simulink model "blockdemo"  (Simulink 7.0)
settings: Solver=FixedStepDiscrete  StartTime=0.0  StopTime=10.0  FixedStep=1  RelTol=1e-3
InitFcn:
  | %% DSPBuilder Start
  | alt_dspbuilder_update_model(bdroot)
  | %% DSPBuilder End
libraries: allblocks_alteradspbuilder2 x12
settings Model: Creator=mjervis  LastModifiedBy=delphick
settings OptimizationCC: BlockReduction=off  BooleanDataType=off  InlineInvariantSignals=on
settings DebuggingCC: SaveWithParameterizedLinksMsg=none  SignalResolutionControl=TryResolveAllWithWarning  SolverPrmCheckMsg=none  MultiTaskDSMMsg=warning  MultiTaskCondExecSysMsg=none
settings HardwareCC: TargetUnknown=on
settings RTWCC: IncludeERTFirstTime=on
settings GRTTargetCC: TargetFcnLib=ansi_tfl_tmw.mat

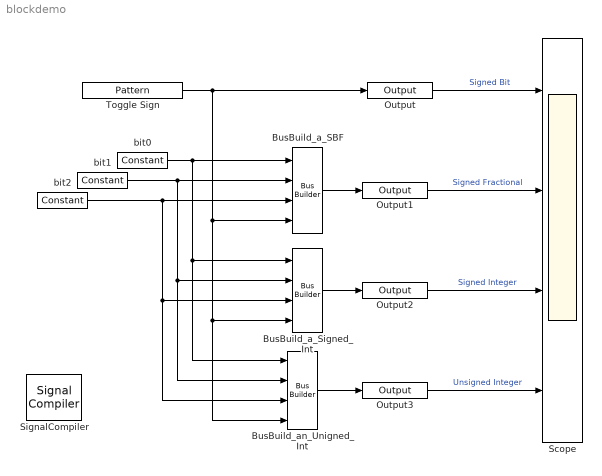
== system blockdemo ==
  BusBuild_a_SBF : allblocks_alteradspbuilder2/Bus Builder  BusType=Signed Fractional  bwl=2  bwr=2  pipeline_display=0
  BusBuild_a_Signed_Int : allblocks_alteradspbuilder2/Bus Builder  BusType=Signed Integer  bwl=4  bwr=0  pipeline_display=0
  BusBuild_an_Unigned_Int : allblocks_alteradspbuilder2/Bus Builder  BusType=Unsigned Integer  bwl=4  bwr=0  pipeline_display=0
  Output : allblocks_alteradspbuilder2/Output  iofile=C:\perforce_workspace81\main\dsp_builder2\Documentation\DesignExamples\Tutorials\UnitBlocks\IOBus\BusBuilder\tb_blockdemo\blockdemo_Output.capture  BusType=Single Bit  bwl=8  bwr=0  externalType=Inferred  PORTTYPE=Output  allowFloatingPointOverride=on  logOutputs=off
  Output1 : allblocks_alteradspbuilder2/Output  iofile=C:\perforce_workspace81\main\dsp_builder2\Documentation\DesignExamples\Tutorials\UnitBlocks\IOBus\BusBuilder\tb_blockdemo\blockdemo_Output1.capture  BusType=Signed Fractional  bwl=2  bwr=2  externalType=Inferred  PORTTYPE=Output  allowFloatingPointOverride=on  logOutputs=off
  Output2 : allblocks_alteradspbuilder2/Output  iofile=C:\perforce_workspace81\main\dsp_builder2\Documentation\DesignExamples\Tutorials\UnitBlocks\IOBus\BusBuilder\tb_blockdemo\blockdemo_Output2.capture  BusType=Signed Integer  bwl=4  bwr=0  externalType=Inferred  PORTTYPE=Output  allowFloatingPointOverride=on  logOutputs=off
  Output3 : allblocks_alteradspbuilder2/Output  iofile=C:\perforce_workspace81\main\dsp_builder2\Documentation\DesignExamples\Tutorials\UnitBlocks\IOBus\BusBuilder\tb_blockdemo\blockdemo_Output3.capture  BusType=Unsigned Integer  bwl=4  bwr=0  externalType=Inferred  PORTTYPE=Output  allowFloatingPointOverride=on  logOutputs=off
  Scope : Scope  NumInputPorts=4
      settings: YMin=-1~-2~-8~0  YMax=2~1~2~10
  SignalCompiler : allblocks_alteradspbuilder2/Signal Compiler  DeviceFamily=Stratix IV  DeviceName=AUTO  EnableSignalTap=off  SignalTapDepth=128  UseBoardBlock=off  StpUseDefaultClock=on  StpClock=Clock  ExportDir=C:\Documents and Settings\delphick\My Documents\MATLAB
  Toggle Sign : allblocks_alteradspbuilder2/Pattern  Sequence=11110000  SpecifyClock=off  use_ena=off  use_sclr=off
  bit0 : allblocks_alteradspbuilder2/Constant  mask_cst=1  BusType=Single Bit  bwl=8  bwr=0  roundMode=Truncate  satMode=Wrap  SpecifyClock=off  allowFloatingPointOverride=on  logOutputs=off  logFile=C:\perforce_workspace81\main\dsp_builder2\Documentation\DesignExamples\Tutorials\UnitBlocks\IOBus\BusBuilder\tb_blockdemo\blockdemo_bit0.fixedpointlog
  bit1 : allblocks_alteradspbuilder2/Constant  mask_cst=0  BusType=Single Bit  bwl=8  bwr=0  roundMode=Truncate  satMode=Wrap  SpecifyClock=off  allowFloatingPointOverride=on  logOutputs=off  logFile=C:\perforce_workspace81\main\dsp_builder2\Documentation\DesignExamples\Tutorials\UnitBlocks\IOBus\BusBuilder\tb_blockdemo\blockdemo_bit1.fixedpointlog
  bit2 : allblocks_alteradspbuilder2/Constant  mask_cst=0  BusType=Single Bit  bwl=8  bwr=0  roundMode=Truncate  satMode=Wrap  SpecifyClock=off  allowFloatingPointOverride=on  logOutputs=off  logFile=C:\blockdemo_bit2.fixedpointlog
  wires:
  BusBuild_a_SBF/1 -> Output1/1
  BusBuild_a_Signed_Int/1 -> Output2/1
  BusBuild_an_Unigned_Int/1 -> Output3/1
  bit2/1 -> BusBuild_a_Signed_Int/3, BusBuild_an_Unigned_Int/3, BusBuild_a_SBF/3
  bit1/1 -> BusBuild_a_Signed_Int/2, BusBuild_an_Unigned_Int/2, BusBuild_a_SBF/2
  bit0/1 -> BusBuild_a_Signed_Int/1, BusBuild_an_Unigned_Int/1, BusBuild_a_SBF/1
  Toggle Sign/1 -> BusBuild_a_Signed_Int/4, BusBuild_an_Unigned_Int/4, BusBuild_a_SBF/4, Output/1
  Output/1 -> Scope/1  "Signed Bit"
  Output1/1 -> Scope/2  "Signed Fractional"
  Output2/1 -> Scope/3  "Signed Integer"
  Output3/1 -> Scope/4  "Unsigned Integer"
